simulink model "P2PHVDCMMC"  (R2024a)
settings: Solver=FixedStepDiscrete  StartTime=0.0  StopTime=10  RelTol=1e-3
PreLoadFcn:
  | % HVDCMMCInterconnectionParam
StartFcn:
  | tic
StopFcn:
  | toc
values from neighbouring files (symbols this model uses):
  C_PM = 1.758e-3    (= 0.001758)    [P2PHVDCMMCcode.m]
  Cg = 50e-9    (= 5e-08)    [P2PHVDCMMCcode.m]
  Fc = Fnom*3.37    (= 168.5)    [P2PHVDCMMCcode.m]
  Fnom = 50    [P2PHVDCMMCcode.m]
  Ki_Ireg = 6    [P2PHVDCMMCcode.m]
  Ki_Preg = 1.0    (= 1)    [P2PHVDCMMCcode.m]
  Ki_Qreg = 1.0    (= 1)    [P2PHVDCMMCcode.m]
  Ki_VDCreg = 100    [P2PHVDCMMCcode.m]
  Kp_Ireg = 0.6    [P2PHVDCMMCcode.m]
  Kp_Preg = 0.5/3    (= 0.166666666667)    [P2PHVDCMMCcode.m]
  Kp_Qreg = 0.5/3    (= 0.166666666667)    [P2PHVDCMMCcode.m]
  Kp_VDCreg = 4    [P2PHVDCMMCcode.m]
  L_cable = 15e-3    (= 0.015)    [P2PHVDCMMCcode.m]
  Larm = Larm_pu*(Zb_ac/(2*pi*Fnom))    [P2PHVDCMMCcode.m]
  Larm_pu = 0.15    [P2PHVDCMMCcode.m]
  Lff = Larm_pu/2    (= 0.075)    [P2PHVDCMMCcode.m]
  Limits_Ireg = [ 2.0  -2.0]    [P2PHVDCMMCcode.m]
  Limits_Preg = [ 1.2, 0.8 ]    [P2PHVDCMMCcode.m]
  Limits_Qreg = [ 0.25, -0.25 ]    [P2PHVDCMMCcode.m]
  Limits_VDCreg = [ 2.0  -2.0]    [P2PHVDCMMCcode.m]
  Lxfo = 0.12    [P2PHVDCMMCcode.m]
  N = 1    [P2PHVDCMMCcode.m]
  Nb_PM = 36    [P2PHVDCMMCcode.m]
  Pnom = 1000e6    (= 1000000000)    [P2PHVDCMMCcode.m]
  R_cable = 0.5    [P2PHVDCMMCcode.m]
  R_startup = 400    [P2PHVDCMMCcode.m]
  Rarm = Rarm_pu*Zb_ac    [P2PHVDCMMCcode.m]
  Rff = Rarm_pu/2    (= 0.00075)    [P2PHVDCMMCcode.m]
  Rg = 100    [P2PHVDCMMCcode.m]
  Rxfo = 0.003    [P2PHVDCMMCcode.m]
  Slope_Qref = 0.5    [P2PHVDCMMCcode.m]
  Slope_Vdc_ref = Vnom_dc/5    (= 128000)    [P2PHVDCMMCcode.m]
  Ts = Ts_Control    (= 4e-05)    [P2PHVDCMMCcode.m]
  Ts_Control = 40e-6    (= 4e-05)    [P2PHVDCMMCcode.m]
  Ts_Power = 20e-6    (= 2e-05)    [P2PHVDCMMCcode.m]
  Vnom_dc = 640e3    (= 640000)    [P2PHVDCMMCcode.m]
  Vnom_prim = 400e3    (= 400000)    [P2PHVDCMMCcode.m]
  Vnom_sec = 333e3    (= 333000)    [P2PHVDCMMCcode.m]
undefined symbols (not defined in the file or in its folder): DiscIntNeverNeededParam, Discrete, gcbh, HRM, Pcc, S, sps, sps_rtmsupport, spsMeanValueVariableFrequencyModel, spsPLL3phModel, SY3, Tfault
libraries: simulink x38, spsControlledVoltageSourceLib x30, DQsym_Lib x25, spsVoltageMeasurementLib x21, spsIdealSwitchLib x21, powerlib_extras x12, spsSecondOrderFilterLib x12, spsCurrentMeasurementLib x12, spsdq0toabcLib x9, spsMeanLib x8, spsMeanVariableFrequencyLib x8, spsabctodq0Lib x8
(part 3 of 8)

== system P2PHVDCMMC/Control _DQn_rec/Current Regulator (Ireg)2 ==
  note: -----------
      | | Lconv |
      | ------------
  note: <---
  note: -------o
  note: Vconv
  note: ----
  note: -----------
      | | Rconv |
      | -----------
  note: For L >> R :
  note: (Vq_sys - Vq_conv) ~ = - Id * L
  note: (Vd_sys - Vd_conv) ~= + Iq * L
  note: Id positive --> The converter generates active power= P positive
  note: Iq negative --> The converter generates reactive power ("Capacitive mode") = Q positive
  note: Sign Convention: Current going out of the converter = positive current
  note: Current Regulator
      | (with feedforward)
  note: Vq_sys + Id*w*L + Iq*R + deriv(Iq)*L= Vq_conv
  note: Vd_sys + Id*R - Iq*w*L + deriv(Id)*L= Vd_conv
  note: (Note: Derivative terms replaced by PI controllers)
  note: Vsys
  note: o-------
  note: I
  IdIq_ref : Inport  PortDimensions=2
  IdIq : Inport  Port=2  PortDimensions=2
  VdVq : Inport  Port=3  PortDimensions=2
  Freq : Inport  Port=4  PortDimensions=1
  wt : Inport  Port=5  PortDimensions=1
  Vdc : Inport  Port=6  PortDimensions=1
  " (Hz)" : Constant  Value=Vnom_dc  SampleTime=Ts
  Add1 : Sum  Inputs=+++-
  Add3 : Sum  Inputs=++++
  Avoid division by zero1 : Saturate  UpperLimit=Vnom_dc*1.25  LowerLimit=Vnom_dc*0.75
  Constant1 : Constant  Value=Lff  SampleTime=Ts_Control
  Constant2 : Constant  Value=Lff  SampleTime=Ts_Control
  Constant3 : Constant  Value=0  SampleTime=Ts
  Demux{,1..4} (5 alike) : Demux  Outputs=2
  Divide : Product  Inputs=*/
  Divide1 : Product  Inputs=**
  Gain : Gain  Gain=Rff
  Gain1 : Gain  Gain=Rff
  Gain2 : Gain  Gain=[ [0, 1 ,zeros(1,N+2)]; [zeros(1,N+4)];[zeros(1,N+4)]]
  Math Function : Math  Operator=hypot  SignedPower=on
  Mean : spsMeanLib/Mean  Freq=Fnom/3  Vinit=Vnom_dc  Ts=Ts
  Mux : Mux  Inputs=2
  Mux1 : Mux  Inputs=2
  Mux2 : Mux  Inputs=[2 1]
  PI regulator with anti-windup D : Subsystem  DialogController=POWERSYS.PowerSysDialog  mask(Discrete PI Controller){Kp=Kp_Ireg, Ki=Ki_Ireg, Par_Limits=Limits_Ireg, Init=0, Ts=Ts}
      mask prompts: Kp "Proportional gain (Kp):"; Ki "Integral gain (Ki):"; Par_Limits "Output limits: [ Upper   Lower ]"; Init "Output initial value:"; Ts "Sample time:"
      mask help: This block implements a discrete PI controller.
      mask init:
      | UpperLimit=Par_Limits(1);
      | LowerLimit=Par_Limits(2);
      | power_initmask();
      mask Help: This block is part of a subset of blocks in the Extras library that does not have documentation associated with it, other than the block mask description.
      mask Display: disp('PI');
  PI regulator with anti-windup Q : Subsystem  DialogController=POWERSYS.PowerSysDialog  mask(Discrete PI Controller){Kp=Kp_Ireg, Ki=Ki_Ireg, Par_Limits=Limits_Ireg, Init=0, Ts=Ts}
      mask prompts: Kp "Proportional gain (Kp):"; Ki "Integral gain (Ki):"; Par_Limits "Output limits: [ Upper   Lower ]"; Init "Output initial value:"; Ts "Sample time:"
      mask help: This block implements a discrete PI controller.
      mask init:
      | UpperLimit=Par_Limits(1);
      | LowerLimit=Par_Limits(2);
      | power_initmask();
      mask Help: This block is part of a subset of blocks in the Extras library that does not have documentation associated with it, other than the block mask description.
      mask Display: disp('PI');
  Product1 : Product  Inputs=3  RndMeth=Zero
  Product2 : Product  Inputs=3  RndMeth=Zero
  Real-Imag to Complex : RealImagToComplex
  Rtot_pu3 : Gain  Gain=1/Fnom  SaturateOnIntegerOverflow=on  OutDataTypeStr=Inherit: Same as input  ParamDataTypeStr=Inherit: Same as input
  Saturation : Saturate  UpperLimit=Limits_Ireg(1)  LowerLimit=Limits_Ireg(2)
  Sum : Sum  Inputs=|-+
  Sum1 : Sum  Inputs=|-+
  dq0 to abc : spsdq0toabcLib/dq0 to abc  Alignment=90 degrees behind phase A axis
  to-pu : Gain  Gain=1/(Vnom_dc/2*sqrt(3)/sqrt(2)/Vnom_sec)
  Uref_ABC : Outport
  Uref_dq0 : Outport  Port=2
  tag scope: PIdq_dqn_rec=global, m_dqn_rec=global
  wires:
  to-pu/1 -> Saturation/1
  Mux/1 -> Divide1/1
  dq0 to abc/1 -> Uref_ABC/1
  Divide/1 -> Divide1/2
  Mean/1 -> Avoid division by zero1/1
  Divide1/1 -> to-pu/1
  " (Hz)"/1 -> Divide/1
  Vdc/1 -> Mean/1
  Avoid division by zero1/1 -> Divide/2
  Mux1/1 -> [PIdq_dqn_rec]
  Constant3/1 -> Mux2/2
  Mux2/1 -> dq0 to abc/1
  PI regulator with anti-windup D/1(Out) -> [PId], Add1/2
  PI regulator with anti-windup Q/1(Out) -> [PIq], Add3/2
  [Vd] -> Add1/1
  Product1/1 -> Add1/4
  Gain/1 -> Add1/3
  Gain1/1 -> Add3/3
  Product2/1 -> Add3/4
  [Vq] -> Add3/1
  Demux2/1 -> [Id]
  IdIq/1 -> Demux2/1
  [Id_ref] -> Product2/1
  [Iq_ref] -> Gain1/1
  [Iq_ref] -> Product1/1
  [Id_ref] -> Gain/1
  [Id] -> Sum/1
  [Iq] -> Sum1/1
  Demux2/2 -> [Iq]
  [PIq] -> Mux1/2
  [PId] -> Mux1/1
  [w] -> Product1/3
  Constant2/1 -> Product1/2
  [w] -> Product2/3
  Constant1/1 -> Product2/2
  [Iq_ref] -> Sum1/2
  Sum1/1 -> PI regulator with anti-windup Q/1(Error)
  [Id_ref] -> Sum/2
  Sum/1 -> PI regulator with anti-windup D/1(Error)
  VdVq/1 -> Demux3/1
  Demux3/2 -> [Vq]
  Demux3/1 -> [Vd]
  IdIq_ref/1 -> Demux1/1
  Demux1/2 -> [Iq_ref]
  Demux1/1 -> [Id_ref]
  Rtot_pu3/1 -> [w]
  Freq/1 -> Rtot_pu3/1
  Add1/1 -> Mux/1
  Add3/1 -> Mux/2
  wt/1 -> dq0 to abc/2
  Demux4/2 -> Real-Imag to Complex/2
  Demux4/1 -> Real-Imag to Complex/1
  Real-Imag to Complex/1 -> Gain2/1
  Gain2/1 -> Uref_dq0/1
  Math Function/1 -> [m_dqn_rec]
  Demux/1 -> Math Function/1
  Demux/2 -> Math Function/2
  Saturation/1 -> Demux/1, Demux4/1, Mux2/1

== system P2PHVDCMMC/Control _DQn_rec/DC Voltage Regulator (VDCreg) ==
  note: VDC Regulator
  Vdc_meas : Inport  PortDimensions=1
  Vdc_ref : Inport  Port=2  PortDimensions=1
  On : Inport  Port=3  PortDimensions=1
  Discrete-Time Integrator : DiscreteIntegrator  SampleTime=Ts  LimitOutput=on  UpperSaturationLimit=Limits_VDCreg(1)  LowerSaturationLimit=Limits_VDCreg(2)  ICPrevOutput=DiscIntNeverNeededParam  ICPrevScaledInput=DiscIntNeverNeededParam
  Product : Product  RndMeth=Zero
  Product1 : Product  RndMeth=Zero
  Rtot_pu2 : Gain  Gain=1/Vnom_dc  SaturateOnIntegerOverflow=on  OutDataTypeStr=Inherit: Same as input  ParamDataTypeStr=Inherit: Same as input
  Saturation2 : Saturate  UpperLimit=Limits_VDCreg(1)  LowerLimit=Limits_VDCreg(2)  SampleTime=Ts
  Sum : Sum  Inputs=|+-
  Sum6 : Sum  InputSameDT=on  SaturateOnIntegerOverflow=on  SampleTime=Ts  OutDataTypeStr=Inherit: Same as first input
  Switch1 : Switch  Criteria=u2 ~= 0  Threshold=0.5  OutDataTypeStr=double  SaturateOnIntegerOverflow=off  InputSameDT=off
  VdcNom_SM : Constant  Value=Kp_VDCreg
  VdcNom_SM1 : Constant  Value=Ki_VDCreg
  Zero-Order Hold : ZeroOrderHold  SampleTime=Ts
  Id_ref : Outport
  wires:
  Rtot_pu2/1 -> Product/2, Product1/2
  Saturation2/1 -> Id_ref/1
  VdcNom_SM/1 -> Product1/1
  Product/1 -> Discrete-Time Integrator/1
  Product1/1 -> Zero-Order Hold/1
  VdcNom_SM1/1 -> Product/1
  Sum6/1 -> Saturation2/1
  Discrete-Time Integrator/1 -> Sum6/2
  Zero-Order Hold/1 -> Sum6/1
  Vdc_ref/1 -> Sum/2, Switch1/3
  Switch1/1 -> Sum/1
  On/1 -> Switch1/2
  Sum/1 -> Rtot_pu2/1
  Vdc_meas/1 -> Switch1/1

== system P2PHVDCMMC/Control _DQn_rec/PLL, Measurements and Transformation1 ==
  note: Q positive = Converter generates reactive power (Capacitive Mode)
  note: P positive = Converter generates active power (Inverter Mode)
  note: Q (pu) = Vq*Id - Vd*Iq
  note: P (pu) = Vd*Id + Vq*Iq
  Vdq : Inport
  Idq : Inport  Port=2
  Add : Sum  Inputs=1
  Constant1 : Constant  Commented=on  Value=0.0004583
  Demux : Demux  Outputs=2
  Discrete Mean value : powerlib_extras/Discrete Measurements/Discrete  Mean value  Freq=Fnom  Vinit=0  Ts=Ts
  Discrete Mean value1 : powerlib_extras/Discrete Measurements/Discrete  Mean value  Freq=Fnom  Vinit=0  Ts=Ts
  From1 : From  Commented=on  TagVisibility=global
  I->pu2 : Gain  Gain=sqrt(3)*Vnom_sec/sqrt(2)/Pnom  SaturateOnIntegerOverflow=on  OutDataTypeStr=Inherit: Same as input  ParamDataTypeStr=Inherit: Same as input
  MATLAB Function : MATLAB Function  TreatAsAtomicUnit=on
  MATLAB Function1 : MATLAB Function  TreatAsAtomicUnit=on
  MATLAB Function2 : MATLAB Function  Commented=on  TreatAsAtomicUnit=on
  Mux : Mux  Inputs=2
  Mux1 : Mux  Inputs=2
  PLL (3ph) : Subsystem  Commented=on  AncestorBlock=|  DialogController=POWERSYS.PowerSysDialog  LoadFcn=sps_rtmsupport('LoadFcn', gcbh);  StartFcn=sps_rtmsupport('StartFcn', gcbh);  StopFcn=sps_rtmsupport('StopFcn', gcbh);  mask(PLL (3ph)){Fmin=0.9*Fnom, Par_Init=[0, Fnom], ParK=[180, 3200, 1], TcD=1e-4, MaxRateChangeFreq=12, FilterCutOffFreq=25, Ts=Ts, AGC=on}
      | spsPLL3phLib/PLL
      | (3ph)
      mask prompts: Fmin "Minimum frequency (Hz):"; Par_Init "Initial inputs [ Phase (degrees), Frequency (Hz) ]:"; ParK "Regulator gains [ Kp, Ki, Kd ]:"; TcD "Time constant for derivative action (s):"; MaxRateChangeFreq "Maximum rate of change of frequency (Hz/s):"; FilterCutOffFreq "Filter cut-off frequency for frequency measurement (Hz):"; Ts "Sample time:"; AGC "Enable automatic gain control"
      mask help:
      | This Phase Locked Loop (PLL) system can be used  to synchronize on a set of variable frequency, three-phase sinusoidal signals. If the Automatic Gain Control is enabled, the input (phase error) of the PLL regulator is scaled according to the input signals magnitude.
      |
      | For optimal performance, set regulator gains [ Kp Ki  Kd ] = [ 180  3200  1 ] and check the Enable Automatic Gain Control parameter.
      |
      | Input : Vector containing the normalized three-phase signals [Va Vb Vc]
      | Output 1:  Measured frequency (Hz) = w/(2pi)
      | Output 2:  Ramp w.t varying between  0 and 2*pi, synchronized on zero crossings of the fundamental (positive-sequence) of phase A.
      mask init:
      | block=gcb;
      | [WantBlockChoice,Ts,sps] = powericon('PLL3phInit',block,Fmin,Par_Init,ParK,TcD, MaxRateChangeFreq, FilterCutOffFreq, AGC,Ts);
      | powericon('SetInternalModels','set',block,WantBlockChoice);
      settings: CopyFcn=sps_rtmsupport('CopyFcn', gcbh);  DeleteFcn=sps_rtmsupport('DeleteFcn', gcbh);  UndoDeleteFcn=sps_rtmsupport('UndoDeleteFcn', gcbh);  ModelCloseFcn=sps_rtmsupport('ModelCloseFcn', gcbh);  PreSaveFcn=sps_rtmsupport('PreSaveFcn', gcbh);  PostSaveFcn=sps_rtmsupport('PostSaveFcn', gcbh);  NameChangeFcn=sps_rtmsupport('NameChangeFcn', gcbh);  PreCopyFcn=sps_rtmsupport('PreCopyFcn', gcbh);  OpenFcn=sps_rtmsupport('OpenFcn', gcbh, [8]);  CloseFcn=sps_rtmsupport('CloseFcn', gcbh);  PreDeleteFcn=sps_rtmsupport('PreDeleteFcn', gcbh);
      mask Help: helpview(psbhelp);
  PLL (3ph)2 : Subsystem  AncestorBlock=|  DialogController=POWERSYS.PowerSysDialog  LoadFcn=sps_rtmsupport('LoadFcn', gcbh);  StartFcn=sps_rtmsupport('StartFcn', gcbh);  StopFcn=sps_rtmsupport('StopFcn', gcbh);  mask(PLL (3ph)){Fmin=0.9*Fnom, Par_Init=[0, Fnom], ParK=[180, 3200, 1], TcD=1e-4, MaxRateChangeFreq=12, FilterCutOffFreq=25, Ts=Ts, AGC=on}
      | spsPLL3phLib/PLL
      | (3ph)
      mask prompts: Fmin "Minimum frequency (Hz):"; Par_Init "Initial inputs [ Phase (degrees), Frequency (Hz) ]:"; ParK "Regulator gains [ Kp, Ki, Kd ]:"; TcD "Time constant for derivative action (s):"; MaxRateChangeFreq "Maximum rate of change of frequency (Hz/s):"; FilterCutOffFreq "Filter cut-off frequency for frequency measurement (Hz):"; Ts "Sample time:"; AGC "Enable automatic gain control"
      mask help:
      | This Phase Locked Loop (PLL) system can be used  to synchronize on a set of variable frequency, three-phase sinusoidal signals. If the Automatic Gain Control is enabled, the input (phase error) of the PLL regulator is scaled according to the input signals magnitude.
      |
      | For optimal performance, set regulator gains [ Kp Ki  Kd ] = [ 180  3200  1 ] and check the Enable Automatic Gain Control parameter.
      |
      | Input : Vector containing the normalized three-phase signals [Va Vb Vc]
      | Output 1:  Measured frequency (Hz) = w/(2pi)
      | Output 2:  Ramp w.t varying between  0 and 2*pi, synchronized on zero crossings of the fundamental (positive-sequence) of phase A.
      mask init:
      | block=gcb;
      | [WantBlockChoice,Ts,sps] = powericon('PLL3phInit',block,Fmin,Par_Init,ParK,TcD, MaxRateChangeFreq, FilterCutOffFreq, AGC,Ts);
      | powericon('SetInternalModels','set',block,WantBlockChoice);
      settings: CopyFcn=sps_rtmsupport('CopyFcn', gcbh);  DeleteFcn=sps_rtmsupport('DeleteFcn', gcbh);  UndoDeleteFcn=sps_rtmsupport('UndoDeleteFcn', gcbh);  ModelCloseFcn=sps_rtmsupport('ModelCloseFcn', gcbh);  PreSaveFcn=sps_rtmsupport('PreSaveFcn', gcbh);  PostSaveFcn=sps_rtmsupport('PostSaveFcn', gcbh);  NameChangeFcn=sps_rtmsupport('NameChangeFcn', gcbh);  PreCopyFcn=sps_rtmsupport('PreCopyFcn', gcbh);  OpenFcn=sps_rtmsupport('OpenFcn', gcbh, [8]);  CloseFcn=sps_rtmsupport('CloseFcn', gcbh);  PreDeleteFcn=sps_rtmsupport('PreDeleteFcn', gcbh);
      mask Help: helpview(psbhelp);
  Product : Product  RndMeth=Zero
  Product1 : Product  RndMeth=Zero
  Rate Transition3 : RateTransition  OutPortSampleTime=Ts_Control
  Second-Order Filter2 : spsSecondOrderFilterLib/Second-Order Filter  FilterType=Lowpass  Fo=Fn_filter  Zeta=Zeta_filter  Ts=Ts  Initialize=off  Vac_Init="[0,  0,  60]"  Vdc_Init=0  PlotResponse=off  FreqRange=[0, 500, 1]
  Second-Order Filter3 : spsSecondOrderFilterLib/Second-Order Filter  FilterType=Lowpass  Fo=Fn_filter  Zeta=Zeta_filter  Ts=Ts  Initialize=off  Vac_Init="[0,  0,  60]"  Vdc_Init=0  PlotResponse=off  FreqRange=[0, 500, 1]
  Selector3 : Selector  InputPortWidth=2  IndexOptions=Index vector (dialog)  Indices=[2 1]  OutputSizes=1
  Subtract : Sum  Inputs=+-
  Sum : Sum  Inputs=|+-
  V->pu1 : Gain  Gain=1/(Vnom_sec/sqrt(3)*sqrt(2))  SaturateOnIntegerOverflow=on  OutDataTypeStr=Inherit: Same as input  ParamDataTypeStr=Inherit: Same as input
  Freq : Outport
  wt : Outport  Port=2
  VdVq : Outport  Port=3
  IdIq : Outport  Port=4
  P : Outport  Port=5
  Q : Outport  Port=6
  wires:
  Idq/1 -> I->pu2/1
  PLL (3ph)2/2(wt) -> Sum/1, wt/1
  Vdq/1 -> V->pu1/1
  PLL (3ph)2/1(Freq) -> Freq/1
  Subtract/1 -> Discrete Mean value1/1
  Add/1 -> Discrete Mean value/1
  Demux/2 -> Subtract/2
  Demux/1 -> Subtract/1
  Product1/1 -> Demux/1
  Product/1 -> Add/1
  Discrete Mean value/1 -> P/1
  Discrete Mean value1/1 -> Q/1
  Selector3/1 -> Product1/1
  Second-Order Filter2/1 -> Selector3/1, Product/1, VdVq/1
  Second-Order Filter3/1 -> Product/2, Product1/2, IdIq/1
  MATLAB Function/1(d) -> Mux/1
  Sum/1 -> MATLAB Function1/2(wt), MATLAB Function/2(wt)
  MATLAB Function/2(q) -> Mux/2
  Mux/1 -> Second-Order Filter2/1
  V->pu1/1 -> PLL (3ph)2/1(DQ), MATLAB Function/1(DQ)
  Mux1/1 -> Second-Order Filter3/1
  MATLAB Function1/1(d) -> Mux1/1
  I->pu2/1 -> MATLAB Function1/1(DQ)
  MATLAB Function1/2(q) -> Mux1/2
  Rate Transition3/1 -> Sum/2
  [wt0] -> Rate Transition3/1

== system P2PHVDCMMC/Control _DQn_rec/Reactive Power Regulator ==
  note: P (pu) = Vd*Id + Vq*Iq (Zero-sequence is not taken into account)
  note: Q (pu) = Vq*Id - Vd*Iq (valid only for balanced & harmonics-free values)
  note: If PLL sync on Vprim --> Vq=0 --> Id = P/Vd et Iq = -1.0 * Q/Vd
  note: Reactive Power Regulator
  VdVq_mes : Inport  PortDimensions=2
  Qmes : Inport  Port=2  PortDimensions=1
  On : Inport  Port=3  PortDimensions=1
  Qref : Inport  Port=4  PortDimensions=1
  Add2 : Sum
  Discrete Mean value1 : powerlib_extras/Discrete Measurements/Discrete  Mean value  Freq=Fnom  Vinit=0  Ts=Ts
  Discrete-Time Integrator : DiscreteIntegrator  SampleTime=Ts  LimitOutput=on  UpperSaturationLimit=Limits_Qreg(1)  LowerSaturationLimit=Limits_Qreg(2)  ICPrevOutput=DiscIntNeverNeededParam  ICPrevScaledInput=DiscIntNeverNeededParam
  Divide : Product  Inputs=*/
  Product : Product  RndMeth=Zero
  Product1 : Product  RndMeth=Zero
  Rtot_pu1 : Gain  Gain=-1  SaturateOnIntegerOverflow=on  OutDataTypeStr=Inherit: Same as input  ParamDataTypeStr=Inherit: Same as input
  Rtot_pu2 : Gain  Gain=-1  SaturateOnIntegerOverflow=on  OutDataTypeStr=Inherit: Same as input  ParamDataTypeStr=Inherit: Same as input
  Saturation : Saturate  UpperLimit=Limits_Qreg(1)  LowerLimit=Limits_Qreg(2)
  Saturation1 : Saturate  UpperLimit=2  LowerLimit=1e-6
  Saturation2 : Saturate  UpperLimit=Limits_Qreg(1)  LowerLimit=Limits_Qreg(2)
  Selector : Selector  InputPortWidth=2  IndexOptions=Index vector (dialog)  Indices=[1]  OutputSizes=1
  Sum : Sum  Inputs=|-+
  Sum6 : Sum  InputSameDT=on  SaturateOnIntegerOverflow=on  SampleTime=Ts  OutDataTypeStr=Inherit: Same as first input
  Switch1 : Switch  Criteria=u2 ~= 0  Threshold=0.5  OutDataTypeStr=double  SaturateOnIntegerOverflow=off  InputSameDT=off
  VdcNom_SM : Constant  Value=Kp_Qreg
  VdcNom_SM1 : Constant  Value=Ki_Qreg
  Zero-Order Hold : ZeroOrderHold  SampleTime=Ts
  Iq_ref : Outport
  wires:
  Qref/1 -> Sum/2, Switch1/3, Divide/1
  Qmes/1 -> Sum/1
  VdVq_mes/1 -> Selector/1
  Selector/1 -> Discrete Mean value1/1
  Divide/1 -> Rtot_pu2/1
  Saturation1/1 -> Divide/2
  Discrete Mean value1/1 -> Saturation1/1
  Zero-Order Hold/1 -> Sum6/1
  Discrete-Time Integrator/1 -> Sum6/2
  VdcNom_SM1/1 -> Product/1
  VdcNom_SM/1 -> Product1/1
  Product1/1 -> Zero-Order Hold/1
  Product/1 -> Discrete-Time Integrator/1
  Add2/1 -> Saturation/1
  On/1 -> Switch1/2
  Sum/1 -> Switch1/1
  Switch1/1 -> Product/2, Product1/2
  Sum6/1 -> Saturation2/1
  Rtot_pu1/1 -> Add2/1
  Rtot_pu2/1 -> Add2/2
  Saturation/1 -> Iq_ref/1
  Saturation2/1 -> Rtot_pu1/1

== system P2PHVDCMMC/Controllers2/Active Power Regulator (Preg) ==
  note: Active Power Regulator
  Pmeas : Inport  PortDimensions=1
  Pref : Inport  Port=2  PortDimensions=1  SampleTime=Ts
  On : Inport  Port=3  PortDimensions=1  SampleTime=Ts
  Discrete-Time Integrator : DiscreteIntegrator  InitialCondition=1  SampleTime=Ts  LimitOutput=on  UpperSaturationLimit=Limits_Preg(1)  LowerSaturationLimit=Limits_Preg(2)  ICPrevOutput=DiscIntNeverNeededParam  ICPrevScaledInput=DiscIntNeverNeededParam
  Product : Product  RndMeth=Zero
  Product1 : Product  RndMeth=Zero
  Product2 : Product
  Saturation2 : Saturate  UpperLimit=Limits_Preg(1)  LowerLimit=Limits_Preg(2)  SampleTime=Ts
  Sum : Sum  Inputs=|+-
  Sum6 : Sum  InputSameDT=on  SaturateOnIntegerOverflow=on  SampleTime=Ts  OutDataTypeStr=Inherit: Same as first input
  Switch1 : Switch  Criteria=u2 ~= 0  Threshold=0.5  OutDataTypeStr=double  SaturateOnIntegerOverflow=off  InputSameDT=off
  VdcNom_SM : Constant  Value=Kp_Preg  SampleTime=Ts
  VdcNom_SM1 : Constant  Value=Ki_Preg  SampleTime=Ts
  VdcNom_SM2 : Constant  Value=Vnom_dc  SampleTime=Ts
  Zero-Order Hold : ZeroOrderHold  SampleTime=Ts
  Vdc_ref : Outport  SampleTime=Ts
  wires:
  Product2/1 -> Vdc_ref/1
  VdcNom_SM2/1 -> Product2/2
  Pmeas/1 -> Switch1/1
  On/1 -> Switch1/2
  Switch1/1 -> Sum/1
  Pref/1 -> Switch1/3, Sum/2
  Zero-Order Hold/1 -> Sum6/1
  Discrete-Time Integrator/1 -> Sum6/2
  Sum6/1 -> Saturation2/1
  VdcNom_SM1/1 -> Product/1
  Product1/1 -> Zero-Order Hold/1
  Product/1 -> Discrete-Time Integrator/1
  VdcNom_SM/1 -> Product1/1
  Saturation2/1 -> Product2/1
  Sum/1 -> Product1/2, Product/2

== system P2PHVDCMMC/Controllers2/Current Regulator (Ireg) ==
  note: -----------
      | | Lconv |
      | ------------
  note: <---
  note: -------o
  note: Vconv
  note: ----
  note: -----------
      | | Rconv |
      | -----------
  note: For L >> R :
  note: (Vq_sys - Vq_conv) ~ = - Id * L
  note: (Vd_sys - Vd_conv) ~= + Iq * L
  note: Id positive --> The converter generates active power= P positive
  note: Iq negative --> The converter generates reactive power ("Capacitive mode") = Q positive
  note: Sign Convention: Current going out of the converter = positive current
  note: Current Regulator
      | (with feedforward)
  note: Vq_sys + Id*w*L + Iq*R + deriv(Iq)*L= Vq_conv
  note: Vd_sys + Id*R - Iq*w*L + deriv(Id)*L= Vd_conv
  note: (Note: Derivative terms replaced by PI controllers)
  note: Vsys
  note: o-------
  note: I
  IdIq_ref : Inport  PortDimensions=2
  IdIq : Inport  Port=2  PortDimensions=2
  VdVq : Inport  Port=3  PortDimensions=2
  Freq : Inport  Port=4  PortDimensions=1
  wt : Inport  Port=5  PortDimensions=1
  Vdc : Inport  Port=6  PortDimensions=1
  " (Hz)" : Constant  Value=Vnom_dc  SampleTime=Ts
  Add1 : Sum  Inputs=+++-
  Add3 : Sum  Inputs=++++
  Avoid division by zero1 : Saturate  UpperLimit=Vnom_dc*1.25  LowerLimit=Vnom_dc*0.75
  Constant1 : Constant  Value=Lff  SampleTime=Ts_Control
  Constant2 : Constant  Value=Lff  SampleTime=Ts_Control
  Constant3 : Constant  Value=0  SampleTime=Ts
  Demux{,1..3} (4 alike) : Demux  Outputs=2
  Divide : Product  Inputs=*/
  Divide1 : Product  Inputs=**
  Gain : Gain  Gain=Rff
  Gain1 : Gain  Gain=Rff
  Math Function : Math  Operator=hypot  SignedPower=on
  Mean : spsMeanLib/Mean  Freq=Fnom/3  Vinit=Vnom_dc  Ts=Ts
  Mux : Mux  Inputs=2
  Mux1 : Mux  Inputs=2
  Mux2 : Mux  Inputs=[2 1]
  PI regulator with anti-windup D : Subsystem  DialogController=POWERSYS.PowerSysDialog  mask(Discrete PI Controller){Kp=Kp_Ireg, Ki=Ki_Ireg, Par_Limits=Limits_Ireg, Init=0, Ts=Ts}
      mask prompts: Kp "Proportional gain (Kp):"; Ki "Integral gain (Ki):"; Par_Limits "Output limits: [ Upper   Lower ]"; Init "Output initial value:"; Ts "Sample time:"
      mask help: This block implements a discrete PI controller.
      mask init:
      | UpperLimit=Par_Limits(1);
      | LowerLimit=Par_Limits(2);
      | power_initmask();
      mask Help: This block is part of a subset of blocks in the Extras library that does not have documentation associated with it, other than the block mask description.
      mask Display: disp('PI');
  PI regulator with anti-windup Q : Subsystem  DialogController=POWERSYS.PowerSysDialog  mask(Discrete PI Controller){Kp=Kp_Ireg, Ki=Ki_Ireg, Par_Limits=Limits_Ireg, Init=0, Ts=Ts}
      mask prompts: Kp "Proportional gain (Kp):"; Ki "Integral gain (Ki):"; Par_Limits "Output limits: [ Upper   Lower ]"; Init "Output initial value:"; Ts "Sample time:"
      mask help: This block implements a discrete PI controller.
      mask init:
      | UpperLimit=Par_Limits(1);
      | LowerLimit=Par_Limits(2);
      | power_initmask();
      mask Help: This block is part of a subset of blocks in the Extras library that does not have documentation associated with it, other than the block mask description.
      mask Display: disp('PI');
  Product1 : Product  Inputs=3  RndMeth=Zero
  Product2 : Product  Inputs=3  RndMeth=Zero
  Rtot_pu3 : Gain  Gain=1/Fnom  SaturateOnIntegerOverflow=on  OutDataTypeStr=Inherit: Same as input  ParamDataTypeStr=Inherit: Same as input
  Saturation : Saturate  UpperLimit=Limits_Ireg(1)  LowerLimit=Limits_Ireg(2)
  Scope : Scope
  Sum : Sum  Inputs=|-+
  Sum1 : Sum  Inputs=|-+
  dq0 to abc : spsdq0toabcLib/dq0 to abc  Alignment=90 degrees behind phase A axis
  to-pu : Gain  Gain=1/(Vnom_dc/2*sqrt(3)/sqrt(2)/Vnom_sec)
  Uref_ABC : Outport
  tag scope: PIdq=global, m=global
  wires:
  wt/1 -> dq0 to abc/2
  to-pu/1 -> Saturation/1
  Mux/1 -> Divide1/1
  dq0 to abc/1 -> Uref_ABC/1
  Divide/1 -> Divide1/2
  Mean/1 -> Avoid division by zero1/1
  Divide1/1 -> to-pu/1
  " (Hz)"/1 -> Divide/1
  Vdc/1 -> Mean/1
  Avoid division by zero1/1 -> Divide/2
  Mux1/1 -> [PIdq]
  Constant3/1 -> Mux2/2
  Mux2/1 -> dq0 to abc/1
  Demux/2 -> Math Function/2
  Demux/1 -> Math Function/1
  Math Function/1 -> [m]
  Saturation/1 -> Mux2/1, Demux/1
  PI regulator with anti-windup D/1(Out) -> [PId], Scope/1, Add1/2
  PI regulator with anti-windup Q/1(Out) -> [PIq], Add3/2
  [Vd] -> Add1/1
  Product1/1 -> Add1/4
  Gain/1 -> Add1/3
  Gain1/1 -> Add3/3
  Product2/1 -> Add3/4
  [Vq] -> Add3/1
  Demux2/1 -> [Id]
  IdIq/1 -> Demux2/1
  [Id_ref] -> Product2/1
  [Iq_ref] -> Gain1/1
  [Iq_ref] -> Product1/1
  [Id_ref] -> Gain/1
  [Id] -> Sum/1
  [Iq] -> Sum1/1
  Demux2/2 -> [Iq]
  [PIq] -> Mux1/2
  [PId] -> Mux1/1
  [w] -> Product1/3
  Constant2/1 -> Product1/2
  [w] -> Product2/3
  Constant1/1 -> Product2/2
  [Iq_ref] -> Sum1/2
  Sum1/1 -> PI regulator with anti-windup Q/1(Error)
  [Id_ref] -> Sum/2
  Sum/1 -> PI regulator with anti-windup D/1(Error)
  VdVq/1 -> Demux3/1
  Demux3/2 -> [Vq]
  Demux3/1 -> [Vd]
  IdIq_ref/1 -> Demux1/1
  Demux1/2 -> [Iq_ref]
  Demux1/1 -> [Id_ref]
  Rtot_pu3/1 -> [w]
  Freq/1 -> Rtot_pu3/1
  Add1/1 -> Mux/1
  Add3/1 -> Mux/2

== system P2PHVDCMMC/Controllers2/DC Voltage Regulator (VDCreg) ==
  note: VDC Regulator
  Vdc_meas : Inport  PortDimensions=1
  Vdc_ref : Inport  Port=2  PortDimensions=1
  On : Inport  Port=3  PortDimensions=1
  Discrete-Time Integrator : DiscreteIntegrator  SampleTime=Ts  LimitOutput=on  UpperSaturationLimit=Limits_VDCreg(1)  LowerSaturationLimit=Limits_VDCreg(2)  ICPrevOutput=DiscIntNeverNeededParam  ICPrevScaledInput=DiscIntNeverNeededParam
  Product : Product  RndMeth=Zero
  Product1 : Product  RndMeth=Zero
  Rtot_pu2 : Gain  Gain=1/Vnom_dc  SaturateOnIntegerOverflow=on  OutDataTypeStr=Inherit: Same as input  ParamDataTypeStr=Inherit: Same as input
  Saturation2 : Saturate  UpperLimit=Limits_VDCreg(1)  LowerLimit=Limits_VDCreg(2)  SampleTime=Ts
  Sum : Sum  Inputs=|+-
  Sum6 : Sum  InputSameDT=on  SaturateOnIntegerOverflow=on  SampleTime=Ts  OutDataTypeStr=Inherit: Same as first input
  Switch1 : Switch  Criteria=u2 ~= 0  Threshold=0.5  OutDataTypeStr=double  SaturateOnIntegerOverflow=off  InputSameDT=off
  VdcNom_SM : Constant  Value=Kp_VDCreg
  VdcNom_SM1 : Constant  Value=Ki_VDCreg
  Zero-Order Hold : ZeroOrderHold  SampleTime=Ts
  Id_ref : Outport
  wires:
  Rtot_pu2/1 -> Product/2, Product1/2
  Saturation2/1 -> Id_ref/1
  VdcNom_SM/1 -> Product1/1
  Product/1 -> Discrete-Time Integrator/1
  Product1/1 -> Zero-Order Hold/1
  VdcNom_SM1/1 -> Product/1
  Sum6/1 -> Saturation2/1
  Discrete-Time Integrator/1 -> Sum6/2
  Zero-Order Hold/1 -> Sum6/1
  Vdc_ref/1 -> Sum/2, Switch1/3
  Switch1/1 -> Sum/1
  On/1 -> Switch1/2
  Sum/1 -> Rtot_pu2/1
  Vdc_meas/1 -> Switch1/1

== system P2PHVDCMMC/Controllers2/PLL, Measurements and Transformation ==
  note: P (pu) = Vd*Id + Vq*Iq
  note: Q (pu) = Vq*Id - Vd*Iq
  note: P positive = Converter generates active power (Inverter Mode)
  note: Q positive = Converter generates reactive power (Capacitive Mode)
  Vabc : Inport  PortDimensions=3
  Iabc : Inport  Port=2  PortDimensions=3
  Add : Sum  Inputs=1
  Demux : Demux  Outputs=2
  Discrete Mean value : powerlib_extras/Discrete Measurements/Discrete  Mean value  Freq=Fnom  Vinit=0  Ts=Ts
  Discrete Mean value1 : powerlib_extras/Discrete Measurements/Discrete  Mean value  Freq=Fnom  Vinit=0  Ts=Ts
  I->pu2 : Gain  Gain=sqrt(3)*Vnom_sec/sqrt(2)/Pnom  SaturateOnIntegerOverflow=on  OutDataTypeStr=Inherit: Same as input  ParamDataTypeStr=Inherit: Same as input
  PLL (3ph) : spsPLL3phLib/PLL (3ph)  Fmin=0.9*Fnom  Par_Init=[0, Fnom]  ParK=[180, 3200, 1]  TcD=1e-4  MaxRateChangeFreq=12  FilterCutOffFreq=25  Ts=Ts  AGC=on
  Product : Product  RndMeth=Zero
  Product1 : Product  RndMeth=Zero
  Second-Order Filter : spsSecondOrderFilterLib/Second-Order Filter  FilterType=Lowpass  Fo=Fn_filter  Zeta=Zeta_filter  Ts=Ts  Initialize=off  Vac_Init="[0,  0,  60]"  Vdc_Init=0  PlotResponse=off  FreqRange=[0, 500, 1]
  Second-Order Filter1 : spsSecondOrderFilterLib/Second-Order Filter  FilterType=Lowpass  Fo=Fn_filter  Zeta=Zeta_filter  Ts=Ts  Initialize=off  Vac_Init="[0,  0,  60]"  Vdc_Init=0  PlotResponse=off  FreqRange=[0, 500, 1]
  Selector3 : Selector  InputPortWidth=2  IndexOptions=Index vector (dialog)  Indices=[2 1]  OutputSizes=1
  Selector4 : Selector  InputPortWidth=3  IndexOptions=Index vector (dialog)  Indices=[1 2]  OutputSizes=1
  Selector5 : Selector  InputPortWidth=3  IndexOptions=Index vector (dialog)  Indices=[1 2]  OutputSizes=1
  Subtract : Sum  Inputs=+-
  V->pu1 : Gain  Gain=1/(Vnom_sec/sqrt(3)*sqrt(2))  SaturateOnIntegerOverflow=on  OutDataTypeStr=Inherit: Same as input  ParamDataTypeStr=Inherit: Same as input
  abc to dq0 : spsabctodq0Lib/abc to dq0  Alignment=90 degrees behind phase A axis
  abc to dq1 : spsabctodq0Lib/abc to dq0  Alignment=90 degrees behind phase A axis
  Freq : Outport
  wt : Outport  Port=2
  VdVq : Outport  Port=3
  IdIq : Outport  Port=4
  P : Outport  Port=5
  Q : Outport  Port=6
  wires:
  Selector3/1 -> Product1/1
  Discrete Mean value1/1 -> Q/1
  Discrete Mean value/1 -> P/1
  Second-Order Filter/1 -> VdVq/1, Product/1, Selector3/1
  Second-Order Filter1/1 -> IdIq/1, Product1/2, Product/2
  Product/1 -> Add/1
  Product1/1 -> Demux/1
  Demux/1 -> Subtract/1
  Demux/2 -> Subtract/2
  Add/1 -> Discrete Mean value/1
  Subtract/1 -> Discrete Mean value1/1
  abc to dq0/1 -> Selector4/1
  PLL (3ph)/1 -> Freq/1
  V->pu1/1 -> abc to dq0/1, PLL (3ph)/1
  Vabc/1 -> V->pu1/1
  PLL (3ph)/2 -> wt/1, abc to dq1/2, abc to dq0/2
  Iabc/1 -> I->pu2/1
  abc to dq1/1 -> Selector5/1
  I->pu2/1 -> abc to dq1/1
  Selector4/1 -> Second-Order Filter/1
  Selector5/1 -> Second-Order Filter1/1

== system P2PHVDCMMC/Controllers2/PWM Generators & Calculation of number of inserted modules (Nin) and number of blocked module (Nbl) ==
  Uref_ABC : Inport  PortDimensions=3
  Block : Inport  Port=2
  Add{,7..11} (6 alike) : Sum  Inputs=1
  Constant{,1..5} (6 alike) : Constant  Value=0
  Constant6 : Constant  Value=[ 0, 36 ]
  Demux1 : Demux  Outputs=3
  Demux2 : Demux  Outputs=3
  Gain1 : Gain  Gain=-1
  Mux{,1..5} (6 alike) : Mux  Inputs=2
  PWM Gen1 : Subsystem  mask(PWM generator for half-bridge MMC){n=Nb_PM, Fc=Fc, Ts=Ts_Power}
      mask prompts: n "Number of half-bridges"; Fc "Carriers frequency (Hz)"; Ts "Sample time (s)"
      mask init:
      | Tc=1/Fc;
      |         Pc= [ 0:360/n:360-360/n]*pi/180;
      |         Offset=Pc/(2*pi);
      |         Offset_Cr=Pc/(2*pi)*Tc;
      |         p=0;
      |         for m=1:2:2*n
      |             p=p+1;
      |             SelectPulsesPS(m)=p;
      |             SelectPulsesPS(m+1)=p+n;
      |         end
  PWM Gen2 : Subsystem  mask(PWM generator for half-bridge MMC){n=Nb_PM, Fc=Fc, Ts=Ts_Power}
      mask prompts: n "Number of half-bridges"; Fc "Carriers frequency (Hz)"; Ts "Sample time (s)"
      mask init: same as P2PHVDCMMC/Controllers2/PWM Generators & Calculation of number of inserted modules (Nin) and number of blocked module (Nbl)/PWM Gen1
  PWM Gen3 : Subsystem  mask(PWM generator for half-bridge MMC){n=Nb_PM, Fc=Fc, Ts=Ts_Power}
      mask prompts: n "Number of half-bridges"; Fc "Carriers frequency (Hz)"; Ts "Sample time (s)"
      mask init: same as P2PHVDCMMC/Controllers2/PWM Generators & Calculation of number of inserted modules (Nin) and number of blocked module (Nbl)/PWM Gen1
  PWM Gen4 : Subsystem  mask(PWM generator for half-bridge MMC){n=Nb_PM, Fc=Fc, Ts=Ts_Power}
      mask prompts: n "Number of half-bridges"; Fc "Carriers frequency (Hz)"; Ts "Sample time (s)"
      mask init: same as P2PHVDCMMC/Controllers2/PWM Generators & Calculation of number of inserted modules (Nin) and number of blocked module (Nbl)/PWM Gen1
  PWM Gen5 : Subsystem  mask(PWM generator for half-bridge MMC){n=Nb_PM, Fc=Fc, Ts=Ts_Power}
      mask prompts: n "Number of half-bridges"; Fc "Carriers frequency (Hz)"; Ts "Sample time (s)"
      mask init: same as P2PHVDCMMC/Controllers2/PWM Generators & Calculation of number of inserted modules (Nin) and number of blocked module (Nbl)/PWM Gen1
  PWM Gen6 : Subsystem  mask(PWM generator for half-bridge MMC){n=Nb_PM, Fc=Fc, Ts=Ts_Power}
      mask prompts: n "Number of half-bridges"; Fc "Carriers frequency (Hz)"; Ts "Sample time (s)"
      mask init: same as P2PHVDCMMC/Controllers2/PWM Generators & Calculation of number of inserted modules (Nin) and number of blocked module (Nbl)/PWM Gen1
  Selector{,1..5} (6 alike) : Selector  InputPortWidth=72  IndexOptions=Index vector (dialog)  Indices=[1:2:71]  OutputSizes=1
  Switch{,1..5} (6 alike) : Switch  Criteria=u2 ~= 0  SaturateOnIntegerOverflow=off  InputSameDT=off
  Terminator{,1..4} (5 alike) : Terminator
  N_Ap : Outport
  N_Bp : Outport  Port=2
  N_Cp : Outport  Port=3
  N_Am : Outport  Port=4
  N_Bm : Outport  Port=5
  N_Cm : Outport  Port=6
  tag scope: Cr_Ap=global, Uref_Ap=global
  wires:
  PWM Gen4/2(Cr) -> Terminator4/1
  PWM Gen5/2(Cr) -> Terminator2/1
  Uref_ABC/1 -> Gain1/1, Demux1/1
  PWM Gen6/2(Cr) -> Terminator3/1
  PWM Gen2/2(Cr) -> Terminator/1
  Demux2/2 -> PWM Gen2/1(Uref)
  Demux2/1 -> PWM Gen1/1(Uref), [Uref_Ap]
  Gain1/1 -> Demux2/1
  PWM Gen1/2(Cr) -> [Cr_Ap]
  PWM Gen3/2(Cr) -> Terminator1/1
  Selector/1 -> Add/1
  Selector1/1 -> Add7/1
  Selector2/1 -> Add8/1
  Selector3/1 -> Add9/1
  Selector4/1 -> Add10/1
  Selector5/1 -> Add11/1
  Constant/1 -> Mux/2
  Add7/1 -> Mux1/1
  Constant1/1 -> Mux1/2
  Constant5/1 -> Mux5/2
  Switch/1 -> N_Ap/1
  Switch3/1 -> N_Am/1
  Mux1/1 -> Switch1/3
  Constant6/1 -> Switch/1, Switch5/1, Switch4/1, Switch3/1, Switch2/1, Switch1/1
  Constant2/1 -> Mux2/2
  Add9/1 -> Mux3/1
  Add8/1 -> Mux2/1
  Mux/1 -> Switch/3
  Switch1/1 -> N_Bp/1
  Constant4/1 -> Mux4/2
  Switch2/1 -> N_Cp/1
  Switch4/1 -> N_Bm/1
  Add/1 -> Mux/1
  Switch5/1 -> N_Cm/1
  Constant3/1 -> Mux3/2
  Add10/1 -> Mux4/1
  Add11/1 -> Mux5/1
  Block/1 -> Switch/2, Switch1/2, Switch2/2, Switch3/2, Switch4/2, Switch5/2
  Mux3/1 -> Switch3/3
  Mux4/1 -> Switch4/3
  Mux5/1 -> Switch5/3
  Mux2/1 -> Switch2/3
  PWM Gen6/1(P) -> Selector5/1
  PWM Gen5/1(P) -> Selector4/1
  PWM Gen4/1(P) -> Selector3/1
  PWM Gen3/1(P) -> Selector2/1
  PWM Gen2/1(P) -> Selector1/1
  PWM Gen1/1(P) -> Selector/1
  Demux2/3 -> PWM Gen3/1(Uref)
  Demux1/1 -> PWM Gen4/1(Uref)
  Demux1/3 -> PWM Gen6/1(Uref)
  Demux1/2 -> PWM Gen5/1(Uref)

== system P2PHVDCMMC/Controllers2/Reactive Power Regulator ==
  note: Reactive Power Regulator
  note: If PLL sync on Vprim --> Vq=0 --> Id = P/Vd et Iq = -1.0 * Q/Vd
  note: Q (pu) = Vq*Id - Vd*Iq (valid only for balanced & harmonics-free values)
  note: P (pu) = Vd*Id + Vq*Iq (Zero-sequence is not taken into account)
  VdVq_mes : Inport  PortDimensions=2
  Qmes : Inport  Port=2  PortDimensions=1
  Qref : Inport  Port=3  PortDimensions=1
  On : Inport  Port=4  PortDimensions=1
  Add2 : Sum
  Discrete Mean value1 : powerlib_extras/Discrete Measurements/Discrete  Mean value  Freq=Fnom  Vinit=0  Ts=Ts
  Discrete-Time Integrator : DiscreteIntegrator  SampleTime=Ts  LimitOutput=on  UpperSaturationLimit=Limits_Qreg(1)  LowerSaturationLimit=Limits_Qreg(2)  ICPrevOutput=DiscIntNeverNeededParam  ICPrevScaledInput=DiscIntNeverNeededParam
  Divide : Product  Inputs=*/
  Product : Product  RndMeth=Zero
  Product1 : Product  RndMeth=Zero
  Rtot_pu1 : Gain  Gain=-1  SaturateOnIntegerOverflow=on  OutDataTypeStr=Inherit: Same as input  ParamDataTypeStr=Inherit: Same as input
  Rtot_pu2 : Gain  Gain=-1  SaturateOnIntegerOverflow=on  OutDataTypeStr=Inherit: Same as input  ParamDataTypeStr=Inherit: Same as input
  Saturation : Saturate  UpperLimit=Limits_Qreg(1)  LowerLimit=Limits_Qreg(2)
  Saturation1 : Saturate  UpperLimit=2  LowerLimit=1e-6
  Saturation2 : Saturate  UpperLimit=Limits_Qreg(1)  LowerLimit=Limits_Qreg(2)
  Selector : Selector  InputPortWidth=2  IndexOptions=Index vector (dialog)  Indices=[1]  OutputSizes=1
  Sum : Sum  Inputs=|-+
  Sum6 : Sum  InputSameDT=on  SaturateOnIntegerOverflow=on  SampleTime=Ts  OutDataTypeStr=Inherit: Same as first input
  Switch1 : Switch  Criteria=u2 ~= 0  Threshold=0.5  OutDataTypeStr=double  SaturateOnIntegerOverflow=off  InputSameDT=off
  VdcNom_SM : Constant  Value=Kp_Qreg
  VdcNom_SM1 : Constant  Value=Ki_Qreg
  Zero-Order Hold : ZeroOrderHold  SampleTime=Ts
  Iq_ref : Outport
  wires:
  Saturation2/1 -> Rtot_pu1/1
  Saturation/1 -> Iq_ref/1
  Rtot_pu2/1 -> Add2/2
  Rtot_pu1/1 -> Add2/1
  Sum6/1 -> Saturation2/1
  Switch1/1 -> Product1/2, Product/2
  Sum/1 -> Switch1/1
  On/1 -> Switch1/2
  Add2/1 -> Saturation/1
  Product/1 -> Discrete-Time Integrator/1
  Product1/1 -> Zero-Order Hold/1
  VdcNom_SM/1 -> Product1/1
  VdcNom_SM1/1 -> Product/1
  Discrete-Time Integrator/1 -> Sum6/2
  Zero-Order Hold/1 -> Sum6/1
  Discrete Mean value1/1 -> Saturation1/1
  Saturation1/1 -> Divide/2
  Divide/1 -> Rtot_pu2/1
  Selector/1 -> Discrete Mean value1/1
  VdVq_mes/1 -> Selector/1
  Qmes/1 -> Sum/1
  Qref/1 -> Divide/1, Switch1/3, Sum/2

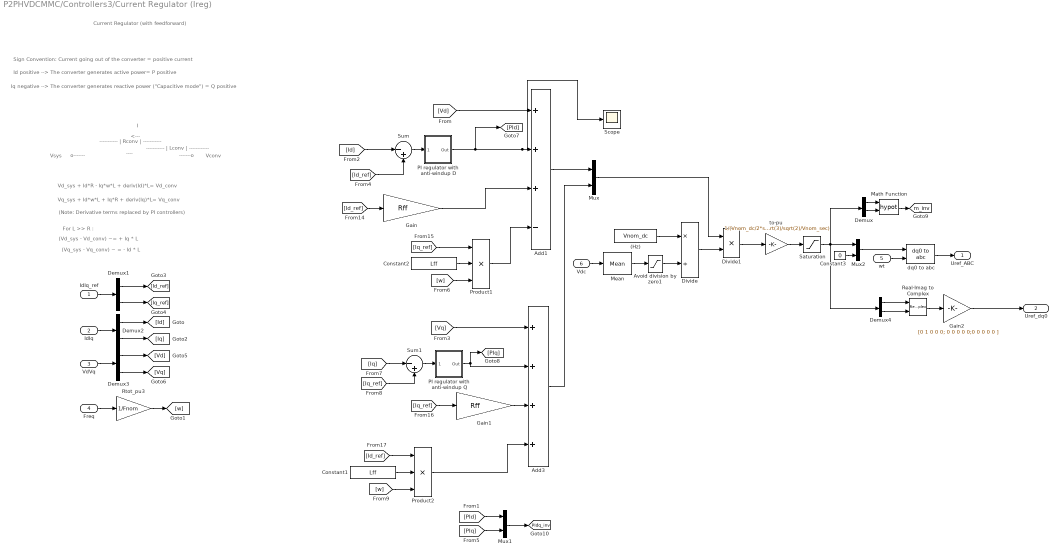
== system P2PHVDCMMC/Controllers3/Current Regulator (Ireg) ==
  note: -----------
      | | Lconv |
      | ------------
  note: <---
  note: -------o
  note: Vconv
  note: ----
  note: -----------
      | | Rconv |
      | -----------
  note: For L >> R :
  note: (Vq_sys - Vq_conv) ~ = - Id * L
  note: (Vd_sys - Vd_conv) ~= + Iq * L
  note: Id positive --> The converter generates active power= P positive
  note: Iq negative --> The converter generates reactive power ("Capacitive mode") = Q positive
  note: Sign Convention: Current going out of the converter = positive current
  note: Current Regulator
      | (with feedforward)
  note: Vq_sys + Id*w*L + Iq*R + deriv(Iq)*L= Vq_conv
  note: Vd_sys + Id*R - Iq*w*L + deriv(Id)*L= Vd_conv
  note: (Note: Derivative terms replaced by PI controllers)
  note: Vsys
  note: o-------
  note: I
  IdIq_ref : Inport  PortDimensions=2
  IdIq : Inport  Port=2  PortDimensions=2
  VdVq : Inport  Port=3  PortDimensions=2
  Freq : Inport  Port=4  PortDimensions=1
  wt : Inport  Port=5  PortDimensions=1
  Vdc : Inport  Port=6  PortDimensions=1
  " (Hz)" : Constant  Value=Vnom_dc  SampleTime=Ts
  Add1 : Sum  Inputs=+++-
  Add3 : Sum  Inputs=++++
  Avoid division by zero1 : Saturate  UpperLimit=Vnom_dc*1.25  LowerLimit=Vnom_dc*0.75
  Constant1 : Constant  Value=Lff  SampleTime=Ts_Control
  Constant2 : Constant  Value=Lff  SampleTime=Ts_Control
  Constant3 : Constant  Value=0  SampleTime=Ts
  Demux{,1..4} (5 alike) : Demux  Outputs=2
  Divide : Product  Inputs=*/
  Divide1 : Product  Inputs=**
  Gain : Gain  Gain=Rff
  Gain1 : Gain  Gain=Rff
  Gain2 : Gain  Gain=[0 1 0 0 0; 0 0 0 0 0;0 0 0 0 0 ]
  Math Function : Math  Operator=hypot  SignedPower=on
  Mean : spsMeanLib/Mean  Freq=Fnom/3  Vinit=Vnom_dc  Ts=Ts
  Mux : Mux  Inputs=2
  Mux1 : Mux  Inputs=2
  Mux2 : Mux  Inputs=[2 1]
  PI regulator with anti-windup D : Subsystem  DialogController=POWERSYS.PowerSysDialog  mask(Discrete PI Controller){Kp=Kp_Ireg, Ki=Ki_Ireg, Par_Limits=Limits_Ireg, Init=0, Ts=Ts}
      mask prompts: Kp "Proportional gain (Kp):"; Ki "Integral gain (Ki):"; Par_Limits "Output limits: [ Upper   Lower ]"; Init "Output initial value:"; Ts "Sample time:"
      mask help: This block implements a discrete PI controller.
      mask init:
      | UpperLimit=Par_Limits(1);
      | LowerLimit=Par_Limits(2);
      | power_initmask();
      mask Help: This block is part of a subset of blocks in the Extras library that does not have documentation associated with it, other than the block mask description.
      mask Display: disp('PI');
  PI regulator with anti-windup Q : Subsystem  DialogController=POWERSYS.PowerSysDialog  mask(Discrete PI Controller){Kp=Kp_Ireg, Ki=Ki_Ireg, Par_Limits=Limits_Ireg, Init=0, Ts=Ts}
      mask prompts: Kp "Proportional gain (Kp):"; Ki "Integral gain (Ki):"; Par_Limits "Output limits: [ Upper   Lower ]"; Init "Output initial value:"; Ts "Sample time:"
      mask help: This block implements a discrete PI controller.
      mask init:
      | UpperLimit=Par_Limits(1);
      | LowerLimit=Par_Limits(2);
      | power_initmask();
      mask Help: This block is part of a subset of blocks in the Extras library that does not have documentation associated with it, other than the block mask description.
      mask Display: disp('PI');
  Product1 : Product  Inputs=3  RndMeth=Zero
  Product2 : Product  Inputs=3  RndMeth=Zero
  Real-Imag to Complex : RealImagToComplex
  Rtot_pu3 : Gain  Gain=1/Fnom  SaturateOnIntegerOverflow=on  OutDataTypeStr=Inherit: Same as input  ParamDataTypeStr=Inherit: Same as input
  Saturation : Saturate  UpperLimit=Limits_Ireg(1)  LowerLimit=Limits_Ireg(2)
  Scope : Scope
  Sum : Sum  Inputs=|-+
  Sum1 : Sum  Inputs=|-+
  dq0 to abc : spsdq0toabcLib/dq0 to abc  Alignment=90 degrees behind phase A axis
  to-pu : Gain  Gain=1/(Vnom_dc/2*sqrt(3)/sqrt(2)/Vnom_sec)
  Uref_ABC : Outport
  Uref_dq0 : Outport  Port=2
  tag scope: PIdq_inv=global, m_inv=global
  wires:
  wt/1 -> dq0 to abc/2
  to-pu/1 -> Saturation/1
  Mux/1 -> Divide1/1
  dq0 to abc/1 -> Uref_ABC/1
  Divide/1 -> Divide1/2
  Mean/1 -> Avoid division by zero1/1
  Divide1/1 -> to-pu/1
  " (Hz)"/1 -> Divide/1
  Vdc/1 -> Mean/1
  Avoid division by zero1/1 -> Divide/2
  Mux1/1 -> [PIdq_inv]
  Constant3/1 -> Mux2/2
  Mux2/1 -> dq0 to abc/1
  Demux/2 -> Math Function/2
  Demux/1 -> Math Function/1
  Math Function/1 -> [m_inv]
  PI regulator with anti-windup D/1(Out) -> [PId], Scope/1, Add1/2
  PI regulator with anti-windup Q/1(Out) -> [PIq], Add3/2
  [Vd] -> Add1/1
  Product1/1 -> Add1/4
  Gain/1 -> Add1/3
  Gain1/1 -> Add3/3
  Product2/1 -> Add3/4
  [Vq] -> Add3/1
  Demux2/1 -> [Id]
  IdIq/1 -> Demux2/1
  [Id_ref] -> Product2/1
  [Iq_ref] -> Gain1/1
  [Iq_ref] -> Product1/1
  [Id_ref] -> Gain/1
  [Id] -> Sum/1
  [Iq] -> Sum1/1
  Demux2/2 -> [Iq]
  [PIq] -> Mux1/2
  [PId] -> Mux1/1
  [w] -> Product1/3
  Constant2/1 -> Product1/2
  [w] -> Product2/3
  Constant1/1 -> Product2/2
  [Iq_ref] -> Sum1/2
  Sum1/1 -> PI regulator with anti-windup Q/1(Error)
  [Id_ref] -> Sum/2
  Sum/1 -> PI regulator with anti-windup D/1(Error)
  VdVq/1 -> Demux3/1
  Demux3/2 -> [Vq]
  Demux3/1 -> [Vd]
  IdIq_ref/1 -> Demux1/1
  Demux1/2 -> [Iq_ref]
  Demux1/1 -> [Id_ref]
  Rtot_pu3/1 -> [w]
  Freq/1 -> Rtot_pu3/1
  Add1/1 -> Mux/1
  Add3/1 -> Mux/2
  Saturation/1 -> Demux/1, Demux4/1, Mux2/1
  Gain2/1 -> Uref_dq0/1
  Real-Imag to Complex/1 -> Gain2/1
  Demux4/1 -> Real-Imag to Complex/1
  Demux4/2 -> Real-Imag to Complex/2

== system P2PHVDCMMC/Controllers3/PLL, Measurements and Transformation ==
  note: P (pu) = Vd*Id + Vq*Iq
  note: Q (pu) = Vq*Id - Vd*Iq
  note: P positive = Converter generates active power (Inverter Mode)
  note: Q positive = Converter generates reactive power (Capacitive Mode)
  Vabc : Inport  PortDimensions=3
  Iabc : Inport  Port=2  PortDimensions=3
  Add : Sum  Inputs=1
  Demux : Demux  Outputs=2
  Discrete Mean value : powerlib_extras/Discrete Measurements/Discrete  Mean value  Freq=Fnom  Vinit=0  Ts=Ts
  Discrete Mean value1 : powerlib_extras/Discrete Measurements/Discrete  Mean value  Freq=Fnom  Vinit=0  Ts=Ts
  I->pu2 : Gain  Gain=sqrt(3)*Vnom_sec/sqrt(2)/Pnom  SaturateOnIntegerOverflow=on  OutDataTypeStr=Inherit: Same as input  ParamDataTypeStr=Inherit: Same as input
  PLL (3ph) : spsPLL3phLib/PLL (3ph)  Fmin=0.9*Fnom  Par_Init=[0, Fnom]  ParK=[180, 3200, 1]  TcD=1e-4  MaxRateChangeFreq=12  FilterCutOffFreq=25  Ts=Ts  AGC=on
  Product : Product  RndMeth=Zero
  Product1 : Product  RndMeth=Zero
  Second-Order Filter : spsSecondOrderFilterLib/Second-Order Filter  FilterType=Lowpass  Fo=Fn_filter  Zeta=Zeta_filter  Ts=Ts  Initialize=off  Vac_Init="[0,  0,  60]"  Vdc_Init=0  PlotResponse=off  FreqRange=[0, 500, 1]
  Second-Order Filter1 : spsSecondOrderFilterLib/Second-Order Filter  FilterType=Lowpass  Fo=Fn_filter  Zeta=Zeta_filter  Ts=Ts  Initialize=off  Vac_Init="[0,  0,  60]"  Vdc_Init=0  PlotResponse=off  FreqRange=[0, 500, 1]
  Selector3 : Selector  InputPortWidth=2  IndexOptions=Index vector (dialog)  Indices=[2 1]  OutputSizes=1
  Selector4 : Selector  InputPortWidth=3  IndexOptions=Index vector (dialog)  Indices=[1 2]  OutputSizes=1
  Selector5 : Selector  InputPortWidth=3  IndexOptions=Index vector (dialog)  Indices=[1 2]  OutputSizes=1
  Subtract : Sum  Inputs=+-
  V->pu1 : Gain  Gain=1/(Vnom_sec/sqrt(3)*sqrt(2))  SaturateOnIntegerOverflow=on  OutDataTypeStr=Inherit: Same as input  ParamDataTypeStr=Inherit: Same as input
  abc to dq0 : spsabctodq0Lib/abc to dq0  Alignment=90 degrees behind phase A axis
  abc to dq1 : spsabctodq0Lib/abc to dq0  Alignment=90 degrees behind phase A axis
  Freq : Outport
  wt : Outport  Port=2
  VdVq : Outport  Port=3
  IdIq : Outport  Port=4
  P : Outport  Port=5
  Q : Outport  Port=6
  wires:
  Selector3/1 -> Product1/1
  Discrete Mean value1/1 -> Q/1
  Discrete Mean value/1 -> P/1
  Second-Order Filter/1 -> VdVq/1, Product/1, Selector3/1
  Second-Order Filter1/1 -> IdIq/1, Product1/2, Product/2
  Product/1 -> Add/1
  Product1/1 -> Demux/1
  Demux/1 -> Subtract/1
  Demux/2 -> Subtract/2
  Add/1 -> Discrete Mean value/1
  Subtract/1 -> Discrete Mean value1/1
  abc to dq0/1 -> Selector4/1
  PLL (3ph)/1 -> Freq/1
  V->pu1/1 -> abc to dq0/1, PLL (3ph)/1
  Vabc/1 -> V->pu1/1
  PLL (3ph)/2 -> wt/1, abc to dq1/2, abc to dq0/2
  Iabc/1 -> I->pu2/1
  abc to dq1/1 -> Selector5/1
  I->pu2/1 -> abc to dq1/1
  Selector4/1 -> Second-Order Filter/1
  Selector5/1 -> Second-Order Filter1/1

== system P2PHVDCMMC/Controllers3/Reactive Power Regulator ==
  note: Reactive Power Regulator
  note: If PLL sync on Vprim --> Vq=0 --> Id = P/Vd et Iq = -1.0 * Q/Vd
  note: Q (pu) = Vq*Id - Vd*Iq (valid only for balanced & harmonics-free values)
  note: P (pu) = Vd*Id + Vq*Iq (Zero-sequence is not taken into account)
  VdVq_mes : Inport  PortDimensions=2
  Qmes : Inport  Port=2  PortDimensions=1
  Qref : Inport  Port=3  PortDimensions=1
  On : Inport  Port=4  PortDimensions=1
  Add2 : Sum
  Discrete Mean value1 : powerlib_extras/Discrete Measurements/Discrete  Mean value  Freq=Fnom  Vinit=0  Ts=Ts
  Discrete-Time Integrator : DiscreteIntegrator  SampleTime=Ts  LimitOutput=on  UpperSaturationLimit=Limits_Qreg(1)  LowerSaturationLimit=Limits_Qreg(2)  ICPrevOutput=DiscIntNeverNeededParam  ICPrevScaledInput=DiscIntNeverNeededParam
  Divide : Product  Inputs=*/
  Product : Product  RndMeth=Zero
  Product1 : Product  RndMeth=Zero
  Rtot_pu1 : Gain  Gain=-1  SaturateOnIntegerOverflow=on  OutDataTypeStr=Inherit: Same as input  ParamDataTypeStr=Inherit: Same as input
  Rtot_pu2 : Gain  Gain=-1  SaturateOnIntegerOverflow=on  OutDataTypeStr=Inherit: Same as input  ParamDataTypeStr=Inherit: Same as input
  Saturation : Saturate  UpperLimit=Limits_Qreg(1)  LowerLimit=Limits_Qreg(2)
  Saturation1 : Saturate  UpperLimit=2  LowerLimit=1e-6
  Saturation2 : Saturate  UpperLimit=Limits_Qreg(1)  LowerLimit=Limits_Qreg(2)
  Selector : Selector  InputPortWidth=2  IndexOptions=Index vector (dialog)  Indices=[1]  OutputSizes=1
  Sum : Sum  Inputs=|-+
  Sum6 : Sum  InputSameDT=on  SaturateOnIntegerOverflow=on  SampleTime=Ts  OutDataTypeStr=Inherit: Same as first input
  Switch1 : Switch  Criteria=u2 ~= 0  Threshold=0.5  OutDataTypeStr=double  SaturateOnIntegerOverflow=off  InputSameDT=off
  VdcNom_SM : Constant  Value=Kp_Qreg
  VdcNom_SM1 : Constant  Value=Ki_Qreg
  Zero-Order Hold : ZeroOrderHold  SampleTime=Ts
  Iq_ref : Outport
  wires:
  Saturation2/1 -> Rtot_pu1/1
  Saturation/1 -> Iq_ref/1
  Rtot_pu2/1 -> Add2/2
  Rtot_pu1/1 -> Add2/1
  Sum6/1 -> Saturation2/1
  Switch1/1 -> Product1/2, Product/2
  Sum/1 -> Switch1/1
  On/1 -> Switch1/2
  Add2/1 -> Saturation/1
  Product/1 -> Discrete-Time Integrator/1
  Product1/1 -> Zero-Order Hold/1
  VdcNom_SM/1 -> Product1/1
  VdcNom_SM1/1 -> Product/1
  Discrete-Time Integrator/1 -> Sum6/2
  Zero-Order Hold/1 -> Sum6/1
  Discrete Mean value1/1 -> Saturation1/1
  Saturation1/1 -> Divide/2
  Divide/1 -> Rtot_pu2/1
  Selector/1 -> Discrete Mean value1/1
  VdVq_mes/1 -> Selector/1
  Qmes/1 -> Sum/1
  Qref/1 -> Divide/1, Switch1/3, Sum/2
